simulink model "CaseBoffline"  (R2014b)
settings: Solver=ode45  SolverMode=SingleTasking  StartTime=0.0  StopTime=100  RelTol=1e-3
libraries: simulink x1
settings Model: CovMetricSettings=dwe  CovHtmlReporting=off  covSaveCumulativeToWorkspaceVar=off  CovSaveSingleToWorkspaceVar=off  CovExternalEMLEnable=on  CovSFcnEnable=on  Creator=Tartan  LastModifiedBy=Tartan
settings DataIOCC: LimitDataPoints=off  SaveFormat=StructureWithTime
settings DebuggingCC: SolverPrmCheckMsg=none  FrameProcessingCompatibilityMsg=error  SFUnexpectedBacktrackingDiag=error  SFNoUnconditionalDefaultTransitionDiag=error
settings HardwareCC: ProdBitPerPointer=64  ProdLargestAtomicFloat=Float  ProdIntDivRoundTo=Zero  ProdEndianess=LittleEndian  ProdHWDeviceType=Specified
settings ModelReferenceCC: PropagateSignalLabelsOutOfModel=on
settings GRTTargetCC: TargetLangStandard=C99 (ISO)  GeneratePreprocessorConditionals=Use local settings

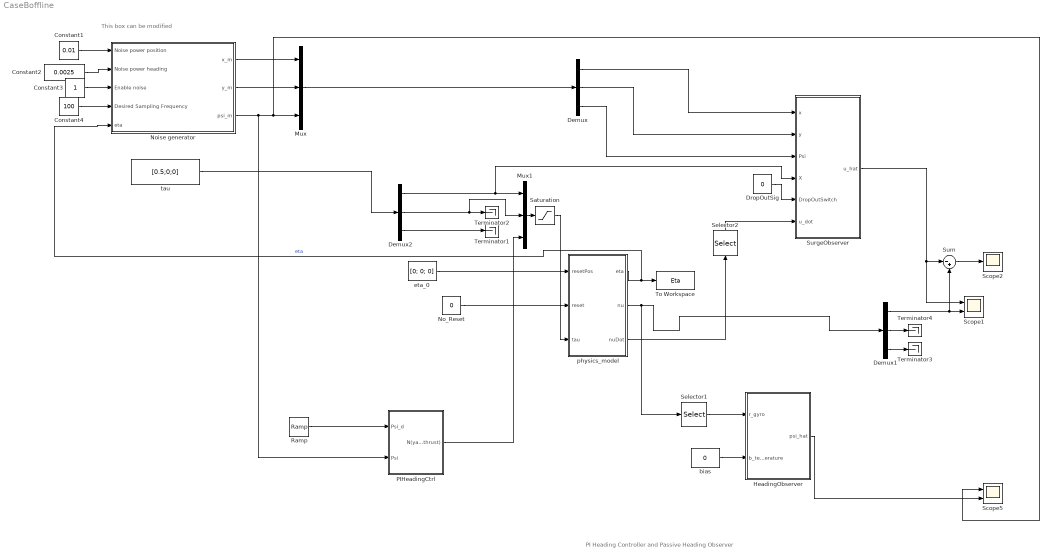
== system CaseBoffline ==
  note: PI Heading Controller and Passive Heading Observer
  note: This box can be modified
  Constant1 : Constant  Value=0.01
  Constant2 : Constant  Value=0.0025
  Constant3 : Constant
  Constant4 : Constant  Value=100
  Demux : Demux  Outputs=3
  Demux1 : Demux  Outputs=3
  Demux2 : Demux  Outputs=3
  DropOutSig : Constant  Value=0
  HeadingObserver : Subsystem
  Mux : Mux  Inputs=3
  Mux1 : Mux  Inputs=3
  No_Reset : Constant  Value=0
  Noise generator : Subsystem
  PIHeadingCtrl : Subsystem
  Ramp : simulink/Sources/Ramp  slope=0  start=0  X0=0.2
  Saturation : Saturate  UpperLimit=[1.03;2.5;0.98]  LowerLimit=-[1.03;2.5;0.98]
  Scope1 : Scope  NumInputPorts=2
      settings: TimeRange=auto  ShowLegends=on  MaxDataPoints=5000  SaveToWorkspace=off  YMin=-9.38388~-0.05285  YMax=6.31386~0.47565  SampleTime=-1
  Scope2 : Scope
      settings: TimeRange=auto  MaxDataPoints=5000  SaveToWorkspace=off  SaveName=ScopeData2  YMin=-0.12775  YMax=0.63196  SampleTime=-1
  Scope5 : Scope  NumInputPorts=2
      settings: TimeRange=auto  ShowLegends=on  MaxDataPoints=5000  SaveToWorkspace=off  YMin=-1.67893~-5  YMax=2.5547~5  SampleTime=-1
  Selector1 : Selector  InputPortWidth=3  IndexOptions=Index vector (dialog)  Indices=[3]  OutputSizes=1
  Selector2 : Selector  InputPortWidth=3  IndexOptions=Index vector (dialog)  Indices=[1]  OutputSizes=1
  Sum : Sum  Inputs=|-+
  SurgeObserver : Subsystem
  Terminator{1..4} (4 alike) : Terminator
  To Workspace : ToWorkspace  VariableName=Eta  SampleTime=-1
  bias : Constant  Value=0
  eta_0 : Constant  Value=[0; 0; 0]
  physics_model : Subsystem
  tau : Constant  Value=[0.5;0;0]
  wires:
  Demux/1 -> SurgeObserver/1(x)
  Demux/2 -> SurgeObserver/2("y ")
  Demux/3 -> SurgeObserver/3(Psi)
  SurgeObserver/1(u_hat) -> Sum/1, Scope1/1
  eta_0/1 -> physics_model/1(resetPos)
  tau/1 -> Demux2/1
  physics_model/3(nuDot) -> Selector2/1
  Demux2/3 -> Terminator1/1
  Demux2/2 -> Mux1/2, Terminator2/1
  physics_model/2(nu) -> Selector1/1, Demux1/1
  Demux1/3 -> Terminator3/1
  Demux1/2 -> Terminator4/1
  Demux1/1 -> Sum/2, Scope1/2
  Sum/1 -> Scope2/1
  Constant2/1 -> Noise generator/2(Noise power heading)
  Constant1/1 -> Noise generator/1(Noise power position)
  Constant3/1 -> Noise generator/3(Enable noise)
  Constant4/1 -> Noise generator/4(Desired Sampling Frequency)
  Noise generator/1(x_m) -> Mux/1
  Noise generator/2(y_m) -> Mux/2
  Noise generator/3(psi_m) -> PIHeadingCtrl/2(Psi), Scope5/1, Mux/3
  physics_model/1(eta) -> To Workspace/1, Noise generator/5(eta)  "eta"
  Mux/1 -> Demux/1
  HeadingObserver/1(psi_hat) -> Scope5/2
  Selector1/1 -> HeadingObserver/1(r_gyro)
  bias/1 -> HeadingObserver/2(b_temperature)
  Demux2/1 -> SurgeObserver/4(X), Mux1/1
  Mux1/1 -> Saturation/1
  Saturation/1 -> physics_model/3(tau)
  DropOutSig/1 -> SurgeObserver/5(DropOutSwitch)
  Selector2/1 -> SurgeObserver/6(u_dot)
  Ramp/1 -> PIHeadingCtrl/1(Psi_d)
  PIHeadingCtrl/1(N(yaw_thrust)) -> Mux1/3
  No_Reset/1 -> physics_model/2(reset)

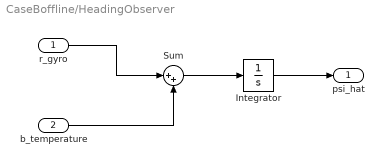
== system CaseBoffline/HeadingObserver ==
  r_gyro : Inport
  b_temperature : Inport  Port=2
  Integrator : Integrator
  Sum : Sum  Inputs=|++
  psi_hat : Outport
  wires:
  Integrator/1 -> psi_hat/1
  r_gyro/1 -> Sum/1
  b_temperature/1 -> Sum/2
  Sum/1 -> Integrator/1

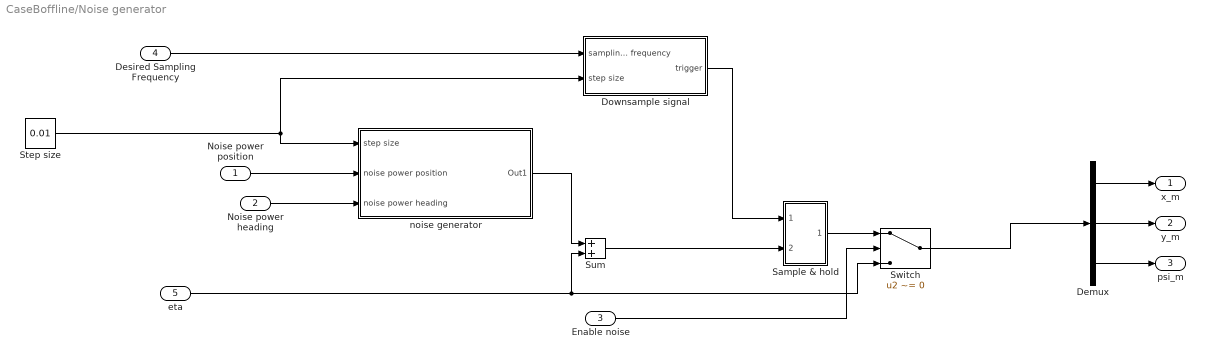
== system CaseBoffline/Noise generator ==
  Noise power position : Inport
  Noise power heading : Inport  Port=2
  Enable noise : Inport  Port=3
  Desired Sampling Frequency : Inport  Port=4
  eta : Inport  Port=5
  Demux : Demux  Outputs=3
  Downsample	signal : Subsystem
  Sample & hold : Subsystem
  Step size : Constant  Value=0.01
  Sum : Sum
  Switch : Switch  Criteria=u2 ~= 0
  noise generator : Subsystem
  x_m : Outport
  y_m : Outport  Port=2
  psi_m : Outport  Port=3
  wires:
  Step size/1 -> Downsample	signal/2(step size), noise generator/1(step size)
  Downsample	signal/1(trigger) -> Sample & hold/1(trigger)
  Desired Sampling Frequency/1 -> Downsample	signal/1(sampling frequency)
  eta/1 -> Sum/2, Switch/3
  Sum/1 -> Sample & hold/2(input)
  Sample & hold/1(output) -> Switch/1
  Noise power position/1 -> noise generator/2(noise power position)
  Noise power heading/1 -> noise generator/3(noise power heading)
  noise generator/1(Out1) -> Sum/1
  Enable noise/1 -> Switch/2
  Switch/1 -> Demux/1
  Demux/3 -> psi_m/1
  Demux/2 -> y_m/1
  Demux/1 -> x_m/1

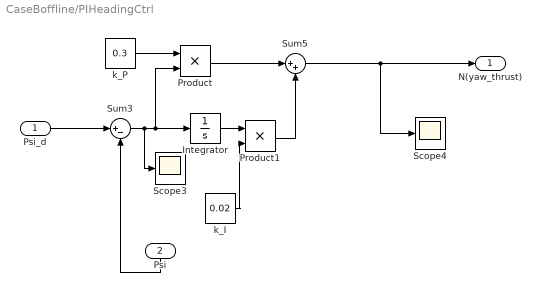
== system CaseBoffline/PIHeadingCtrl ==
  Psi_d : Inport
  Psi : Inport  Port=2
  Integrator : Integrator
  Product : Product
  Product1 : Product
  Scope3 : Scope
      settings: TimeRange=auto  MaxDataPoints=5000  SaveToWorkspace=off  YMin=-2.3547  YMax=1.87893  SampleTime=-1
  Scope4 : Scope
      settings: TimeRange=auto  MaxDataPoints=5000  SaveToWorkspace=off  SaveName=ScopeData2  YMin=-0.68429  YMax=0.51646  SampleTime=-1
  Sum3 : Sum  Inputs=|+-
  Sum5 : Sum  Inputs=|++
  k_I : Constant  Value=0.02
  k_P : Constant  Value=0.3
  N(yaw_thrust) : Outport
  wires:
  Psi/1 -> Sum3/2
  k_P/1 -> Product/1
  Sum3/1 -> Scope3/1, Integrator/1, Product/2
  Product/1 -> Sum5/1
  k_I/1 -> Product1/2
  Product1/1 -> Sum5/2
  Integrator/1 -> Product1/1
  Sum5/1 -> N(yaw_thrust)/1, Scope4/1
  Psi_d/1 -> Sum3/1

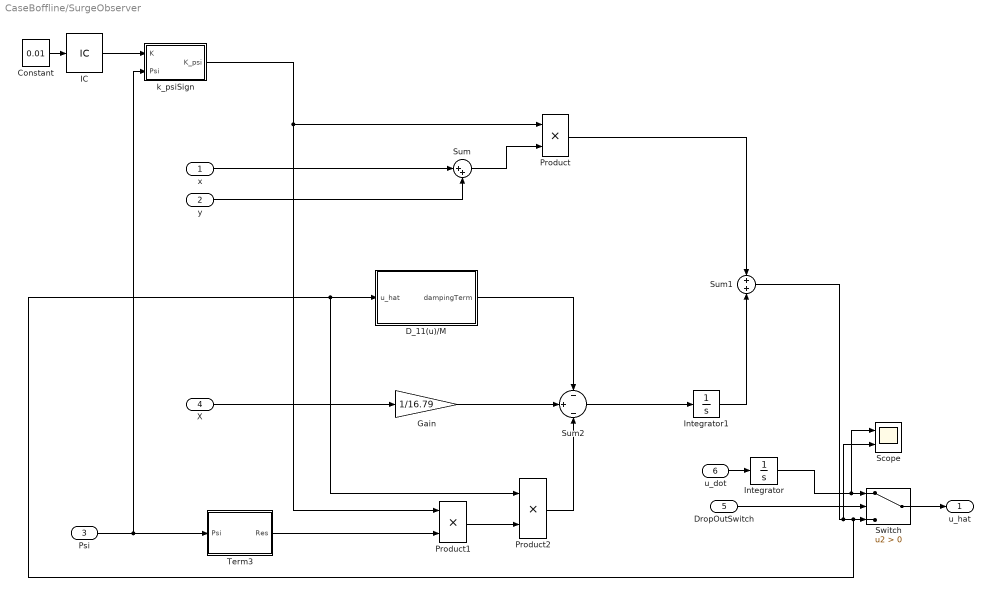
== system CaseBoffline/SurgeObserver ==
  x : Inport
  "y " : Inport  Port=2
  Psi : Inport  Port=3
  X : Inport  Port=4
  DropOutSwitch : Inport  Port=5
  u_dot : Inport  Port=6
  Constant : Constant  Value=0.01
  D_11(u)/M : MATLAB Function  TreatAsAtomicUnit=on
      settings: PermitHierarchicalResolution=ParametersOnly
  Gain : Gain  Gain=1/16.79
  IC : InitialCondition  Value=0.001
  Integrator : Integrator
  Integrator1 : Integrator
  Product : Product
  Product1 : Product
  Product2 : Product
  Scope : Scope  NumInputPorts=2
      settings: TimeRange=auto  ShowLegends=on  MaxDataPoints=5000  SaveToWorkspace=off  SaveName=ScopeData2  YMin=-0.05285~-5  YMax=0.47565~5  SampleTime=-1
  Sum : Sum  Inputs=|++
  Sum1 : Sum  Inputs=+|+
  Sum2 : Sum  Inputs=-|+|-
  Switch : Switch  Criteria=u2 > Threshold
  Term3 : MATLAB Function  TreatAsAtomicUnit=on
      settings: PermitHierarchicalResolution=ParametersOnly
  k_psiSign : MATLAB Function  TreatAsAtomicUnit=on
      settings: PermitHierarchicalResolution=ParametersOnly
  u_hat : Outport
  wires:
  x/1 -> Sum/1
  Sum/1 -> Product/2
  k_psiSign/1(K_psi) -> Product1/1, Product/1
  Product/1 -> Sum1/1
  Sum2/1 -> Integrator1/1
  Integrator1/1 -> Sum1/2
  "y "/1 -> Sum/2
  Sum1/1 -> Scope/2, Product2/1, D_11(u)/M/1(u_hat), Switch/3
  X/1 -> Gain/1
  Gain/1 -> Sum2/2
  Term3/1(Res) -> Product1/2
  Product1/1 -> Product2/2
  D_11(u)/M/1(dampingTerm) -> Sum2/1
  Product2/1 -> Sum2/3
  DropOutSwitch/1 -> Switch/2
  Switch/1 -> u_hat/1
  u_dot/1 -> Integrator/1
  Integrator/1 -> Scope/1, Switch/1
  Psi/1 -> Term3/1(Psi), k_psiSign/2(Psi)
  IC/1 -> k_psiSign/1(K)
  Constant/1 -> IC/1

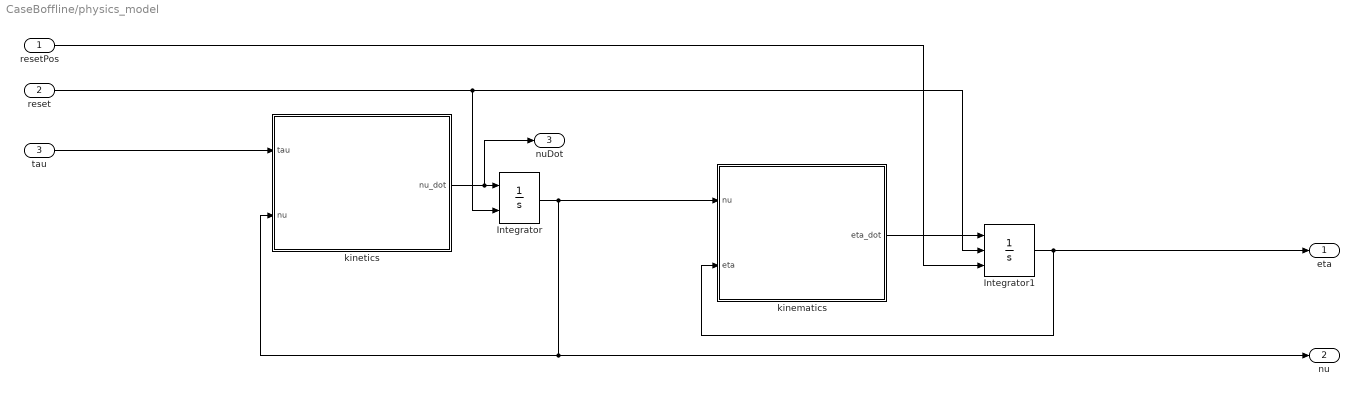
== system CaseBoffline/physics_model ==
  resetPos : Inport
  reset : Inport  Port=2
  tau : Inport  Port=3
  Integrator : Integrator  ExternalReset=rising  InitialCondition=[0 0 0]'
  Integrator1 : Integrator  ExternalReset=rising  InitialConditionSource=external  InitialCondition=[0 0 0]'
  kinematics : MATLAB Function  TreatAsAtomicUnit=on
      settings: PermitHierarchicalResolution=ParametersOnly
  kinetics : MATLAB Function  TreatAsAtomicUnit=on
      settings: PermitHierarchicalResolution=ParametersOnly
  eta : Outport
  nu : Outport  Port=2
  nuDot : Outport  Port=3
  wires:
  kinetics/1(nu_dot) -> nuDot/1, Integrator/1
  Integrator/1 -> nu/1, kinetics/2(nu), kinematics/1(nu)
  kinematics/1(eta_dot) -> Integrator1/1
  Integrator1/1 -> eta/1, kinematics/2(eta)
  reset/1 -> Integrator1/2, Integrator/2
  resetPos/1 -> Integrator1/3
  tau/1 -> kinetics/1(tau)

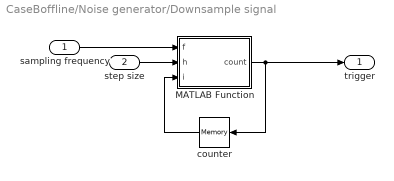
== system CaseBoffline/Noise generator/Downsample	signal ==
  sampling frequency : Inport
  step size : Inport  Port=2
  MATLAB Function : MATLAB Function  TreatAsAtomicUnit=on
      settings: PermitHierarchicalResolution=ParametersOnly
  counter : Memory
  trigger : Outport
  wires:
  sampling frequency/1 -> MATLAB Function/1(f)
  step size/1 -> MATLAB Function/2(h)
  counter/1 -> MATLAB Function/3(i)
  MATLAB Function/1(count) -> counter/1, trigger/1

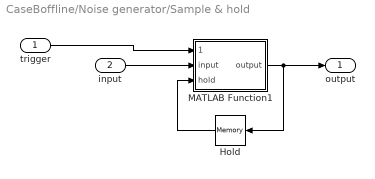
== system CaseBoffline/Noise generator/Sample & hold ==
  trigger : Inport
  input : Inport  Port=2
  Hold : Memory
  MATLAB Function1 : MATLAB Function  TreatAsAtomicUnit=on
      settings: PermitHierarchicalResolution=ParametersOnly
  output : Outport
  wires:
  MATLAB Function1/1(output) -> output/1, Hold/1
  trigger/1 -> MATLAB Function1/1(counter)
  input/1 -> MATLAB Function1/2(input)
  Hold/1 -> MATLAB Function1/3(hold)

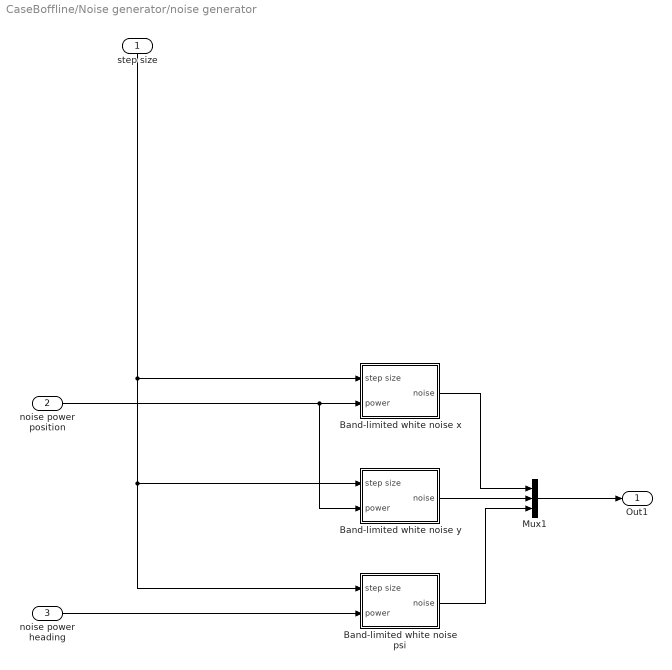
== system CaseBoffline/Noise generator/noise generator ==
  step size : Inport
  noise power position : Inport  Port=2
  noise power heading : Inport  Port=3
  Band-limited white noise psi : Subsystem
  Band-limited white noise x : Subsystem
  Band-limited white noise y : Subsystem
  Mux1 : Mux  Inputs=3
  Out1 : Outport
  wires:
  Mux1/1 -> Out1/1
  step size/1 -> Band-limited white noise x/1(step size), Band-limited white noise psi/1(step size), Band-limited white noise y/1(step size)
  noise power position/1 -> Band-limited white noise y/2(power), Band-limited white noise x/2(power)
  Band-limited white noise x/1(noise) -> Mux1/1
  Band-limited white noise y/1(noise) -> Mux1/2
  Band-limited white noise psi/1(noise) -> Mux1/3
  noise power heading/1 -> Band-limited white noise psi/2(power)

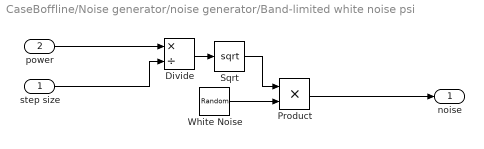
== system CaseBoffline/Noise generator/noise generator/Band-limited white noise psi ==
  step size : Inport
  power : Inport  Port=2
  Divide : Product  Inputs=*/
  Product : Product
  Sqrt : Sqrt  SaturateOnIntegerOverflow=on
  White Noise : RandomNumber  DisableCoverage=on  Seed=9025
  noise : Outport
  wires:
  White Noise/1 -> Product/2
  Product/1 -> noise/1
  step size/1 -> Divide/2
  Divide/1 -> Sqrt/1
  Sqrt/1 -> Product/1
  power/1 -> Divide/1

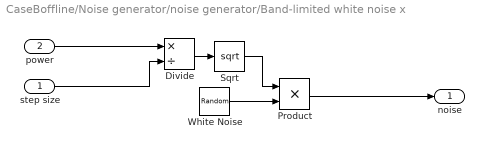
== system CaseBoffline/Noise generator/noise generator/Band-limited white noise x ==
  step size : Inport
  power : Inport  Port=2
  Divide : Product  Inputs=*/
  Product : Product
  Sqrt : Sqrt  SaturateOnIntegerOverflow=on
  White Noise : RandomNumber  DisableCoverage=on  Seed=9024
  noise : Outport
  wires:
  White Noise/1 -> Product/2
  Product/1 -> noise/1
  step size/1 -> Divide/2
  Divide/1 -> Sqrt/1
  Sqrt/1 -> Product/1
  power/1 -> Divide/1

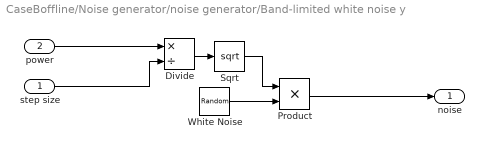
== system CaseBoffline/Noise generator/noise generator/Band-limited white noise y ==
  step size : Inport
  power : Inport  Port=2
  Divide : Product  Inputs=*/
  Product : Product
  Sqrt : Sqrt  SaturateOnIntegerOverflow=on
  White Noise : RandomNumber  DisableCoverage=on  Seed=123
  noise : Outport
  wires:
  White Noise/1 -> Product/2
  Product/1 -> noise/1
  step size/1 -> Divide/2
  Divide/1 -> Sqrt/1
  Sqrt/1 -> Product/1
  power/1 -> Divide/1

== matlab function CaseBoffline/physics_model/kinematics ==
  data: nu input; eta_dot output; eta input
function eta_dot = CSE1_eta_dot(nu,eta)

psi = eta(3);

J = [cos(psi) -sin(psi) 0
     sin(psi) cos(psi)  0
     0        0         1];

eta_dot = J*nu;

== matlab function CaseBoffline/physics_model/kinetics ==
  data: tau input; nu_dot output; nu input
function nu_dot = CSE1_nu_dot_corr(tau,nu)

u   = nu(1);
v   = nu(2);
r   = nu(3);

tau = [tau(1);tau(2);tau(3)];
%% MATRICES

m    = 14.79;   I_z  =  1.7600;   x_g = 0.0375;       % x_g  =  0.0460; % Table B.1


%% Added mass
X_ud  =     -2.0;											% Table B.1
Y_vd =     -10.0;	
N_vd =    -0.0;                                             % Table B.1 guestimate
Y_rd =      -0.0;	
N_rd =    -1.0;                                             % Table B.1

%% Total mass matrix
m_11 = m-X_ud;
m_22 = m-Y_vd;
m_23 = m*x_g-Y_rd;
m_32 = m*x_g-N_vd;
m_33 = I_z-N_rd;

M    = [m_11 0    0
        0    m_22 m_23
        0    m_32 m_33];
	
%% Damping coefficients
% Comments at the end of the lines indicate the old values used.
X_u		= -0.6555;		X_v		= 0;
X_uu 	= 0.3545;		X_vv	= -2.443;
X_uuu 	= -3.787;		X_vvv	= 0;

Y_v		= -1.33; 			Y_r		= -7.250; % Y_r
Y_vv	= -2.776;			Y_rr	= -3.450; % Y_rr
Y_vvv	= -64.91;			Y_rrr	= 0;
						
Y_rv	= -0.805;			Y_vr	= -0.845; % Y_rv, Y_vr

N_v		= 0;				N_r		= -1.900; % N_r
N_vv	= -0.2088;			N_rr	= -0.750; % N_rr
N_vvv	= 0;				N_rrr	= 0;
N_rv	= 0.130;			N_vr	= 0.080; % N_rv, N_vr

%% Correolis matrix

%from ItsLearning
% c_13 = -(m-Y_vd)*v-(m*x_g-Y_rd)*r;
% c_23 = (m-X_ud)*u;
% C    = [0     0     c_13
%         0     0     c_23
%         -c_13 -c_23 0   ];

%From Handbook of Marine Craft Hydr 1st ed pp.120
a1 = X_ud*u;
a2 = Y_vd*v-m*x_g*r;
C    = [0     0     a2
        0     0    -a1
       -a2    a1    0   ];

%% Assembly of the damping matrix
d_11 = -X_u - X_uu*u - X_uuu*u^2;
d_22 = -Y_v - Y_vv*v - Y_vvv*v^2 - Y_rv*abs(r);
d_33 = -N_r - N_rr*abs(r) - N_rrr*r^2 - N_vr*abs(v); % using abs(r)

d_12 = -X_v - X_vv*v - X_vvv*v^2;
d_23 = -Y_r - Y_rr*abs(r) - Y_rrr*r^2 - Y_vr*abs(v);
d_32 = -N_v - N_vv*v - N_vvv*v^2 - N_rv*abs(r);

%From ItsLearning
% D    = [d_11 d_12 0
%         0    d_22 d_23
%         0    d_32 d_33];

%From Feb. 2017 lab manual. Agrees with Handbook of Marine Craft Hydro
D    = [d_11 0    0
        0    d_22 d_23
        0    d_32 d_33];



%% CALCULATION

%nu_dot = M\(tau-(C+D)*nu);
nu_dot = M\(tau-(D)*nu);

== matlab function CaseBoffline/Noise generator/Downsample	signal/MATLAB Function ==
  data: f input; h input; i input; count output
function count = fcn(f,h,i)
%#codegen
sampling_time = 1/f;
if (i+1)*h >= sampling_time
    count = 0;
else
    count = i+1;
end

== matlab function CaseBoffline/Noise generator/Sample & hold/MATLAB Function1 ==
  data: counter input; input input; hold input; output output
function output = fcn(counter,input,hold)
%#codegen

if counter == 0
    output = input;
else
    output = hold;
end

== matlab function CaseBoffline/SurgeObserver/k_psiSign ==
  data: K input; Psi input; K_psi output
function K_psi = fcn(K,Psi)

K_psi=K*sign(cos(Psi)+sin(Psi));


end

== matlab function CaseBoffline/SurgeObserver/D_11(u)//M ==
  data: u_hat input; dampingTerm output
function dampingTerm = fcn(u_hat)
m_11=16.79;
X_u=-0.6555;
X_uu=0.3545;
X_uuu=-3.787;
d_11=-X_u-X_uu*abs(u_hat)-X_uuu*u_hat^2;
dampingTerm=d_11*u_hat/m_11;
end

== matlab function CaseBoffline/SurgeObserver/Term3 ==
  data: Psi input; Res output
function Res = fcn(Psi)

Res=cos(Psi)+sin(Psi);

end
